simulink model "model_knigge_test"  (R2020b)
settings: configuration reference "Configuration" (kept outside this file)
settings Model: Creator=dogukan  LastModifiedBy=dogukan
settings ConfigSetRef: SourceName=Configuration  SourceLocation=Base Workspace

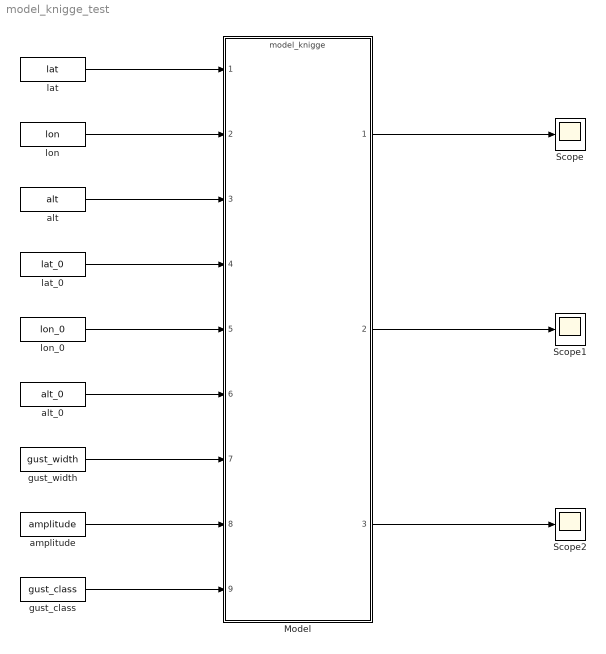
== system model_knigge_test ==
  Model : ModelReference  ModelNameDialog=model_knigge.slx  SimulationMode=Normal  ModelReferenceVersion=1.19
  Scope : Scope
  Scope1 : Scope
  Scope2 : Scope
  alt : FromWorkspace  VariableName=alt
  alt_0 : FromWorkspace  VariableName=alt_0
  amplitude : FromWorkspace  VariableName=amplitude
  gust_class : FromWorkspace  VariableName=gust_class
  gust_width : FromWorkspace  VariableName=gust_width
  lat : FromWorkspace  VariableName=lat
  lat_0 : FromWorkspace  VariableName=lat_0
  lon : FromWorkspace  VariableName=lon
  lon_0 : FromWorkspace  VariableName=lon_0
  wires:
  lon_0/1 -> Model/5
  lat/1 -> Model/1
  lon/1 -> Model/2
  alt/1 -> Model/3
  lat_0/1 -> Model/4
  alt_0/1 -> Model/6
  gust_width/1 -> Model/7
  amplitude/1 -> Model/8
  gust_class/1 -> Model/9
  Model/1 -> Scope/1
  Model/2 -> Scope1/1
  Model/3 -> Scope2/1
